simulink model "two_tanks_model_antiwindup_R2018a"  (R2018a)
settings: Solver=ode23s  StartTime=0.0  StopTime=60*10  FixedStep=0.1  RelTol=1e-3
model workspace (MATLAB code in the model file):
  | A1 = 1;
  | a1 = 0.1*0.1;
  | A2 = A1;
  | a2 = a1;
  | h10 = 1;
  | h20=1;
settings Model: PacingRate=35  Creator=kjartan  LastModifiedBy=kjartan
settings SFSimCC: SimUseLocalCustomCode=on
settings RTWCC: RTWUseLocalCustomCode=on

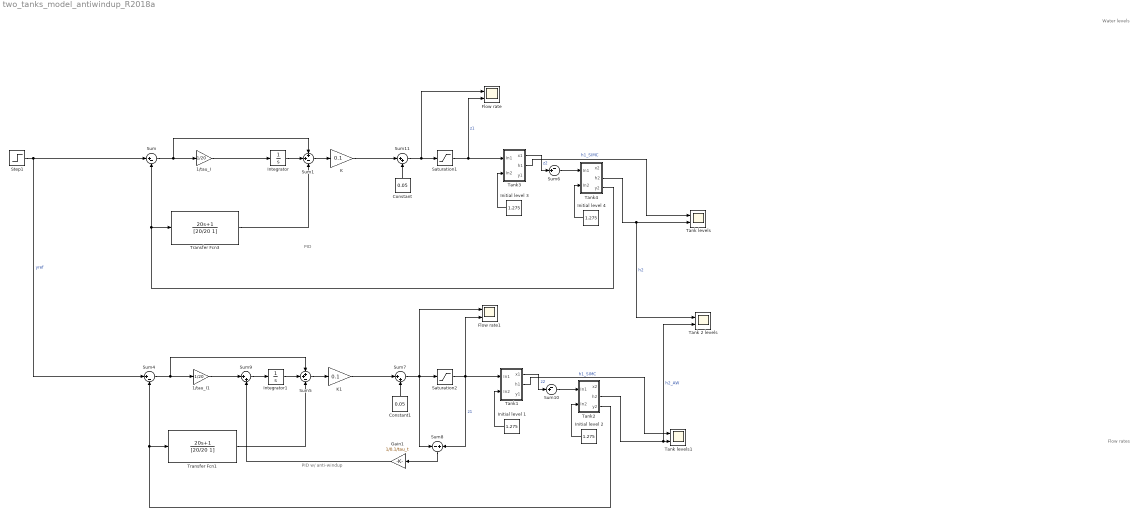
== system two_tanks_model_antiwindup_R2018a ==
  note: PID
  note: Water levels
  note: Flow rates
  note: PID w/ anti-windup
  1/tau_I : Gain  Gain=1/20
  1/tau_I1 : Gain  Gain=1/20
  Constant : Constant  Value=0.05
  Constant1 : Constant  Value=0.05
  Flow rate : Scope  NumInputPorts=2
  Flow rate1 : Scope  NumInputPorts=2
  Gain1 : Gain  Gain=1/0.1/tau_t
  Initial level {1..4} (4 alike) : Constant  Value=1.275
  Integrator : Integrator
  Integrator1 : Integrator
  K : Gain  Gain=0.1
  K1 : Gain  Gain=0.1
  Saturation1 : Saturate  UpperLimit=0.065  LowerLimit=0
  Saturation2 : Saturate  UpperLimit=0.065  LowerLimit=0
  Step1 : Step  Time=120  After=0.4  SampleTime=0
  Sum : Sum  Inputs=|+-
  Sum1 : Sum  Inputs=++-
  Sum10 : Sum  Inputs=-+|
  Sum11 : Sum  Inputs=|++
  Sum4 : Sum  Inputs=|+-
  Sum5 : Sum  Inputs=++-
  Sum6 : Sum  Inputs=-+|
  Sum7 : Sum  Inputs=|++
  Sum8 : Sum  Inputs=-|+
  Sum9 : Sum  Inputs=|++
  Tank 2 levels : Scope  NumInputPorts=2
  Tank levels : Scope  NumInputPorts=2
  Tank levels1 : Scope  NumInputPorts=2
  Tank1 : Subsystem
  Tank2 : Subsystem
  Tank3 : Subsystem
  Tank4 : Subsystem
  Transfer Fcn1 : TransferFcn  Numerator=[20, 1]  Denominator=[20/20 1]
  Transfer Fcn3 : TransferFcn  Numerator=[20, 1]  Denominator=[20/20 1]
  wires:
  Sum1/1 -> K/1
  Initial level 3/1 -> Tank3/2(In2)
  Saturation1/1 -> Flow rate/2, Tank3/1(In1)  "z1"
  Initial level 4/1 -> Tank4/2(In2)
  Step1/1 -> Sum/1, Sum4/1  "yref"
  Sum/1 -> Sum1/1, 1/tau_I/1
  Sum6/1 -> Tank4/1(In1)
  Tank3/1(x1) -> Sum6/2  "z2"
  Tank4/2(h2) -> Tank 2 levels/1, Tank levels/2  "h2"
  K/1 -> Sum11/1
  Sum11/1 -> Flow rate/1, Saturation1/1
  Constant/1 -> Sum11/2
  Transfer Fcn3/1 -> Sum1/3
  Integrator/1 -> Sum1/2
  1/tau_I/1 -> Integrator/1
  Tank3/2(h1) -> Tank levels/1  "h1_SIMC"
  Tank4/3(y2) -> Sum/2, Transfer Fcn3/1
  Sum7/1 -> Flow rate1/1, Sum8/1, Saturation2/1
  Sum5/1 -> K1/1
  Constant1/1 -> Sum7/2
  Transfer Fcn1/1 -> Sum5/3
  Tank1/2(h1) -> Tank levels1/1  "h1_SIMC"
  Tank1/1(x1) -> Sum10/2  "z2"
  Sum9/1 -> Integrator1/1
  Integrator1/1 -> Sum5/2
  Tank2/3(y2) -> Sum4/2, Transfer Fcn1/1
  1/tau_I1/1 -> Sum9/1
  Sum4/1 -> Sum5/1, 1/tau_I1/1
  Saturation2/1 -> Flow rate1/2, Tank1/1(In1), Sum8/2  "z1"
  Initial level 2/1 -> Tank2/2(In2)
  Sum10/1 -> Tank2/1(In1)
  Tank2/2(h2) -> Tank 2 levels/2, Tank levels1/2  "h2_AW"
  Initial level 1/1 -> Tank1/2(In2)
  Sum8/1 -> Gain1/1
  K1/1 -> Sum7/1
  Gain1/1 -> Sum9/2

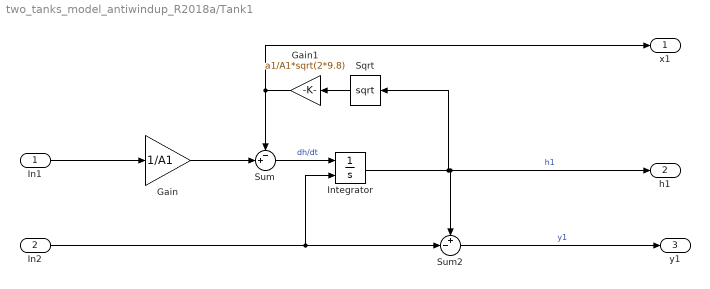
== system two_tanks_model_antiwindup_R2018a/Tank1 ==
  In1 : Inport
  In2 : Inport  Port=2
  Gain : Gain  Gain=1/A1
  Gain1 : Gain  Gain=a1/A1*sqrt(2*9.8)
  Integrator : Integrator  InitialConditionSource=external  InitialCondition=h10  LimitOutput=on  LowerSaturationLimit=0
  Sqrt : Sqrt  SaturateOnIntegerOverflow=on
  Sum : Sum  Inputs=-+|
  Sum2 : Sum  Inputs=+-|
  x1 : Outport  VectorParamsAs1DForOutWhenUnconnected=off
  h1 : Outport  Port=2  VectorParamsAs1DForOutWhenUnconnected=off
  y1 : Outport  Port=3  VectorParamsAs1DForOutWhenUnconnected=off
  wires:
  Gain1/1 -> x1/1, Sum/1
  Gain/1 -> Sum/2
  Sum/1 -> Integrator/1  "dh/dt"
  In1/1 -> Gain/1
  Sum2/1 -> y1/1  "y1"
  Sqrt/1 -> Gain1/1
  Integrator/1 -> Sqrt/1, h1/1, Sum2/1  "h1"
  In2/1 -> Sum2/2, Integrator/2

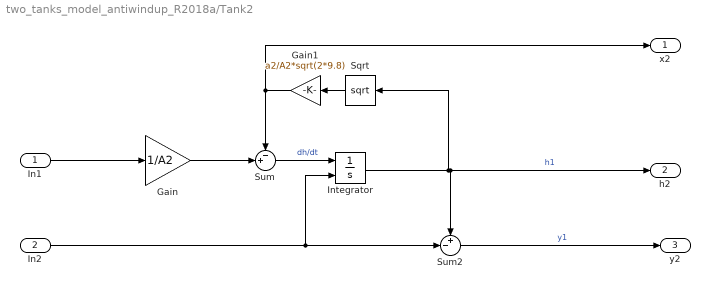
== system two_tanks_model_antiwindup_R2018a/Tank2 ==
  In1 : Inport
  In2 : Inport  Port=2
  Gain : Gain  Gain=1/A2
  Gain1 : Gain  Gain=a2/A2*sqrt(2*9.8)
  Integrator : Integrator  InitialConditionSource=external  InitialCondition=h10  LimitOutput=on  LowerSaturationLimit=0
  Sqrt : Sqrt  SaturateOnIntegerOverflow=on
  Sum : Sum  Inputs=-+|
  Sum2 : Sum  Inputs=+-|
  x2 : Outport  VectorParamsAs1DForOutWhenUnconnected=off
  h2 : Outport  Port=2  VectorParamsAs1DForOutWhenUnconnected=off
  y2 : Outport  Port=3  VectorParamsAs1DForOutWhenUnconnected=off
  wires:
  Gain1/1 -> x2/1, Sum/1
  Gain/1 -> Sum/2
  Sum/1 -> Integrator/1  "dh/dt"
  In1/1 -> Gain/1
  Sum2/1 -> y2/1  "y1"
  Integrator/1 -> Sqrt/1, h2/1, Sum2/1  "h1"
  In2/1 -> Sum2/2, Integrator/2
  Sqrt/1 -> Gain1/1

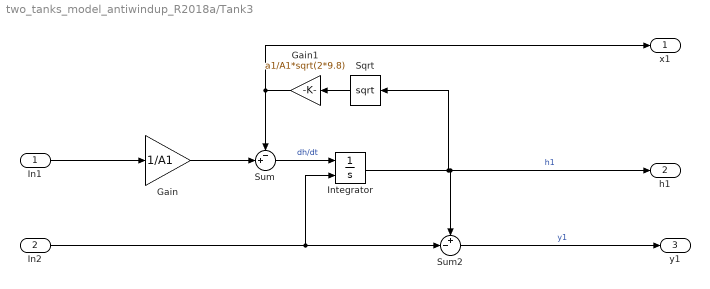
== system two_tanks_model_antiwindup_R2018a/Tank3 ==
  In1 : Inport
  In2 : Inport  Port=2
  Gain : Gain  Gain=1/A1
  Gain1 : Gain  Gain=a1/A1*sqrt(2*9.8)
  Integrator : Integrator  InitialConditionSource=external  InitialCondition=h10  LimitOutput=on  LowerSaturationLimit=0
  Sqrt : Sqrt  SaturateOnIntegerOverflow=on
  Sum : Sum  Inputs=-+|
  Sum2 : Sum  Inputs=+-|
  x1 : Outport  VectorParamsAs1DForOutWhenUnconnected=off
  h1 : Outport  Port=2  VectorParamsAs1DForOutWhenUnconnected=off
  y1 : Outport  Port=3  VectorParamsAs1DForOutWhenUnconnected=off
  wires:
  Gain1/1 -> x1/1, Sum/1
  Gain/1 -> Sum/2
  Sum/1 -> Integrator/1  "dh/dt"
  In1/1 -> Gain/1
  Sum2/1 -> y1/1  "y1"
  Sqrt/1 -> Gain1/1
  Integrator/1 -> Sqrt/1, h1/1, Sum2/1  "h1"
  In2/1 -> Sum2/2, Integrator/2

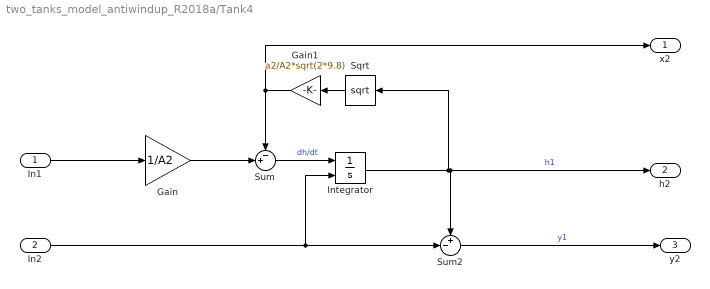
== system two_tanks_model_antiwindup_R2018a/Tank4 ==
  In1 : Inport
  In2 : Inport  Port=2
  Gain : Gain  Gain=1/A2
  Gain1 : Gain  Gain=a2/A2*sqrt(2*9.8)
  Integrator : Integrator  InitialConditionSource=external  InitialCondition=h10  LimitOutput=on  LowerSaturationLimit=0
  Sqrt : Sqrt  SaturateOnIntegerOverflow=on
  Sum : Sum  Inputs=-+|
  Sum2 : Sum  Inputs=+-|
  x2 : Outport  VectorParamsAs1DForOutWhenUnconnected=off
  h2 : Outport  Port=2  VectorParamsAs1DForOutWhenUnconnected=off
  y2 : Outport  Port=3  VectorParamsAs1DForOutWhenUnconnected=off
  wires:
  Gain1/1 -> x2/1, Sum/1
  Gain/1 -> Sum/2
  Sum/1 -> Integrator/1  "dh/dt"
  In1/1 -> Gain/1
  Sum2/1 -> y2/1  "y1"
  Integrator/1 -> Sqrt/1, h2/1, Sum2/1  "h1"
  In2/1 -> Sum2/2, Integrator/2
  Sqrt/1 -> Gain1/1
